simulink model "StepperRTM"  (R2021a)
settings: Solver=FixedStepDiscrete  StartTime=0.0  StopTime=Inf  FixedStep=TSampleStepper  MaxStep=1e-3  RelTol=1e-3  EnableMultiTasking=on
settings Model: SimulationMode=external  ExtModeTrigDuration=8  Creator=lu  LastModifiedBy=lu
settings SolverCC: AlgebraicLoopSolver=TrustRegion  AutoInsertRateTranBlk=on
settings OptimizationCC: DefaultUnderspecifiedDataType=single  PassReuseOutputArgsAs=Individual arguments  MaxStackSize=1024  DenormalBehavior=FlushToZero  EfficientTunableParamExpr=on
settings DebuggingCC: ParameterTunabilityLossMsg=error  SFMachineParentedDataDiag=warning
settings HardwareCC: ProdBitPerChar=16  ProdBitPerInt=16  ProdBitPerPointer=32  ProdBitPerSizeT=32  ProdBitPerPtrDiffT=32  ProdLargestAtomicInteger=Integer  ProdLargestAtomicFloat=None  ProdWordSize=16  ProdLongLongMode=on  ProdHWDeviceType=Texas Instruments->C2000
settings ModelReferenceCC: ModelReferenceNumInstancesAllowed=Single
settings SFSimCC: MATLABDynamicMemAlloc=off
settings RTWCC: SystemTargetFile=ert.tlc  HardwareBoard=TI Piccolo F28004x  GenCodeOnly=on  TemplateMakefile=ert_default_tmf  GenerateReport=on  Toolchain=Texas Instruments Code Composer Studio (C2000)  IncludeHyperlinkInReport=on  LaunchReport=on  GenerateTraceInfo=on  GenerateTraceReport=on  GenerateTraceReportSl=on  GenerateTraceReportSf=on  GenerateTraceReportEml=on  GenerateWebview=on  GenerateCodeMetricsReport=on
settings CodeAppCC: ForceParamTrailComments=on  IgnoreCustomStorageClasses=off  OperatorAnnotations=on  SimulinkDataObjDesc=on  SFDataObjDesc=on  MATLABFcnDesc=on  InsertBlockDesc=on  StateflowObjectComments=on  MATLABSourceComments=on
settings ERTTargetCC: CodeReplacementLibrary=TI C28x  IncludeMdlTerminateFcn=off  SuppressErrorStatus=on  ExtModeTransport=3  ExtModeStaticAllocSize=5000

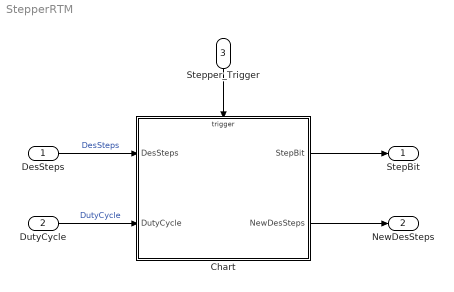
== system StepperRTM ==
  DesSteps : Inport  OutDataTypeStr=uint16
  DutyCycle : Inport  Port=2  OutDataTypeStr=uint16
  Stepper_Trigger : Inport  Port=3  OutDataTypeStr=uint8
  Chart : Stateflow chart  TreatAsAtomicUnit=on
  StepBit : Outport  OutDataTypeStr=uint16
  NewDesSteps : Outport  Port=2  OutDataTypeStr=uint16
  wires:
  Stepper_Trigger/1 -> Chart/Trigger
  DesSteps/1 -> Chart/1(DesSteps)  "DesSteps"
  Chart/1(StepBit) -> StepBit/1
  Chart/2(NewDesSteps) -> NewDesSteps/1
  DutyCycle/1 -> Chart/2(DutyCycle)  "DutyCycle"

== stateflow chart StepperRTM/Chart ==
  settings: sampleTime=TSample
  state Reset
    en: StepBit = 0;
  state Main
    state Idle
      en: StepBit = 0;
    state High
      en: StepBit = 1;
    (default) -> Idle
    Idle -> High : [DesSteps > 0 && after(DutyCycle, Takt)]{NewDesSteps = DesSteps;}
    High -> Idle : [after(DutyCycle,Takt)]{NewDesSteps = (DesSteps - 1);}
  (default) -> Reset
  Reset -> Main : POR
  data: StepBit output uint16; DesSteps input uint16 =0; NewDesSteps output uint16 =0; DutyCycle input uint16
  events: Takt input EITHER_EDGE_EVENT; POR input RISING_EDGE_EVENT
